simulink model "case7"  (R2024b)
settings: Solver=FixedStepAuto  StartTime=0  StopTime=1  FixedStep=1e-7  RelTol=1e-3
values from neighbouring files (symbols this model uses):
  SG_D_1_D = 0.01056    [IEEE9_case_parameters.m]    (also in case1_parameters.m; case2_parameters.m; case3_parameters.m; case4_parameters.m)
  SG_D_1_EnableSaturation = 0    [IEEE9_case_parameters.m]    (also in case1_parameters.m; case2_parameters.m; case3_parameters.m; case4_parameters.m)
  SG_D_1_f0 = 60    [IEEE9_case_parameters.m]    (also in case1_parameters.m; case2_parameters.m; case3_parameters.m; case4_parameters.m)
  SG_D_1_H = 7.5    [IEEE9_case_parameters.m]    (also in case1_parameters.m; case2_parameters.m; case3_parameters.m; case4_parameters.m)
  SG_D_1_K_A = 20    [IEEE9_case_parameters.m]    (also in case1_parameters.m; case2_parameters.m; case3_parameters.m; case4_parameters.m)
  SG_D_1_K_E = 1.000000e+1    (= 10)    [IEEE9_case_parameters.m]    (also in case1_parameters.m; case2_parameters.m; case3_parameters.m; case4_parameters.m)
  SG_D_1_K_F = 2.363    [IEEE9_case_parameters.m]    (also in case1_parameters.m; case2_parameters.m; case3_parameters.m; case4_parameters.m)
  SG_D_1_K_s = 0.5    [IEEE9_case_parameters.m]    (also in case1_parameters.m = 5; case2_parameters.m = 5; case3_parameters.m = 5; case4_parameters.m = 5)
  SG_D_1_R_a = 0.001088    [IEEE9_case_parameters.m]    (also in case1_parameters.m; case2_parameters.m; case3_parameters.m; case4_parameters.m)
  SG_D_1_S_A = 1    [IEEE9_case_parameters.m]    (also in case1_parameters.m; case2_parameters.m; case3_parameters.m; case4_parameters.m)
  SG_D_1_S_B = 0.103    [IEEE9_case_parameters.m]    (also in case1_parameters.m; case2_parameters.m; case3_parameters.m; case4_parameters.m)
  SG_D_1_S_N = 10.659857    [IEEE9_case_parameters.m]    (also in case1_parameters.m; case2_parameters.m; case3_parameters.m; case4_parameters.m)
  SG_D_1_SpeedPara = 200    [IEEE9_case_parameters.m]    (also in case1_parameters.m; case2_parameters.m; case3_parameters.m; case4_parameters.m)
  SG_D_1_T_0 = 0.720173    [IEEE9_case_parameters.m]    (also in case1_parameters.m = 0.755522; case2_parameters.m = 0.808931; case3_parameters.m = 0.869402; case4_parameters.m = 0.729316)
  SG_D_1_T_1 = 0.3    [IEEE9_case_parameters.m]    (also in case1_parameters.m; case2_parameters.m; case3_parameters.m; case4_parameters.m)
  SG_D_1_T_2 = 0.05    [IEEE9_case_parameters.m]    (also in case1_parameters.m; case2_parameters.m; case3_parameters.m; case4_parameters.m)
  SG_D_1_T_3 = 0.02    [IEEE9_case_parameters.m]    (also in case1_parameters.m; case2_parameters.m; case3_parameters.m; case4_parameters.m)
  SG_D_1_T_4 = 0.005    [IEEE9_case_parameters.m]    (also in case1_parameters.m; case2_parameters.m; case3_parameters.m; case4_parameters.m)
  SG_D_1_T_A = 0.02    [IEEE9_case_parameters.m]    (also in case1_parameters.m; case2_parameters.m; case3_parameters.m; case4_parameters.m)
  SG_D_1_T_dd = 8.000000e+0    (= 8)    [IEEE9_case_parameters.m]    (also in case1_parameters.m; case2_parameters.m; case3_parameters.m; case4_parameters.m)
  SG_D_1_T_ddd = 0.04    [IEEE9_case_parameters.m]    (also in case1_parameters.m; case2_parameters.m; case3_parameters.m; case4_parameters.m)
  SG_D_1_T_E = 0.314    [IEEE9_case_parameters.m]    (also in case1_parameters.m; case2_parameters.m; case3_parameters.m; case4_parameters.m)
  SG_D_1_T_F = 0.35    [IEEE9_case_parameters.m]    (also in case1_parameters.m; case2_parameters.m; case3_parameters.m; case4_parameters.m)
  SG_D_1_T_qd = 0.8    [IEEE9_case_parameters.m]    (also in case1_parameters.m; case2_parameters.m; case3_parameters.m; case4_parameters.m)
  SG_D_1_T_qdd = 0.02    [IEEE9_case_parameters.m]    (also in case1_parameters.m; case2_parameters.m; case3_parameters.m; case4_parameters.m)
  SG_D_1_T_speed = 0.1    [IEEE9_case_parameters.m]    (also in case1_parameters.m = 200; case2_parameters.m = 200; case3_parameters.m = 200; case4_parameters.m = 200)
  SG_D_1_T_w = 0.5    [IEEE9_case_parameters.m]    (also in case1_parameters.m; case2_parameters.m; case3_parameters.m; case4_parameters.m)
  SG_D_1_V_ref = 1.990276    [IEEE9_case_parameters.m]    (also in case1_parameters.m = 2.042296; case2_parameters.m = 2.051388; case3_parameters.m = 2.089584; case4_parameters.m = 2.01845)
  SG_D_1_w_ref = 376.991118    [IEEE9_case_parameters.m]    (also in case1_parameters.m; case2_parameters.m; case3_parameters.m; case4_parameters.m)
  SG_D_1_wb = 6.000000e+1    (= 60)    [IEEE9_case_parameters.m]    (also in case1_parameters.m; case2_parameters.m; case3_parameters.m; case4_parameters.m)
  SG_D_1_x_d = 1.9    [IEEE9_case_parameters.m]    (also in case1_parameters.m; case2_parameters.m; case3_parameters.m; case4_parameters.m)
  SG_D_1_x_dd = 0.302    [IEEE9_case_parameters.m]    (also in case1_parameters.m; case2_parameters.m; case3_parameters.m; case4_parameters.m)
  SG_D_1_x_ddd = 0.204    [IEEE9_case_parameters.m]    (also in case1_parameters.m; case2_parameters.m; case3_parameters.m; case4_parameters.m)
  SG_D_1_x_l = 0.05    [IEEE9_case_parameters.m]    (also in case1_parameters.m; case2_parameters.m; case3_parameters.m; case4_parameters.m)
  SG_D_1_x_q = 1.3    [IEEE9_case_parameters.m]    (also in case1_parameters.m; case2_parameters.m; case3_parameters.m; case4_parameters.m)
  SG_D_1_x_qd = 0.5    [IEEE9_case_parameters.m]    (also in case1_parameters.m; case2_parameters.m; case3_parameters.m; case4_parameters.m)
  SG_D_1_x_qdd = 0.3    [IEEE9_case_parameters.m]    (also in case1_parameters.m; case2_parameters.m; case3_parameters.m; case4_parameters.m)
  SG_D_2_D = 0.02    [IEEE9_case_parameters.m]    (also in case1_parameters.m; case2_parameters.m; case3_parameters.m; case4_parameters.m)
  SG_D_2_EnableSaturation = 0    [IEEE9_case_parameters.m]    (also in case1_parameters.m; case2_parameters.m; case3_parameters.m; case4_parameters.m)
  SG_D_2_f0 = 60    [IEEE9_case_parameters.m]    (also in case1_parameters.m; case2_parameters.m; case3_parameters.m; case4_parameters.m)
  SG_D_2_H = 8.000000e+0    (= 8)    [IEEE9_case_parameters.m]    (also in case1_parameters.m; case2_parameters.m; case3_parameters.m; case4_parameters.m)
  SG_D_2_K_A = 20    [IEEE9_case_parameters.m]    (also in case1_parameters.m; case2_parameters.m; case3_parameters.m; case4_parameters.m)
  SG_D_2_K_E = 1.000000e+1    (= 10)    [IEEE9_case_parameters.m]    (also in case1_parameters.m; case2_parameters.m; case3_parameters.m; case4_parameters.m)
  SG_D_2_K_F = 2.363    [IEEE9_case_parameters.m]    (also in case1_parameters.m; case2_parameters.m; case3_parameters.m; case4_parameters.m)
  SG_D_2_K_s = 0.5    [IEEE9_case_parameters.m]    (also in case1_parameters.m = 4; case2_parameters.m = 4; case3_parameters.m = 4; case4_parameters.m = 4)
  SG_D_2_R_a = 0.001088    [IEEE9_case_parameters.m]    (also in case1_parameters.m; case2_parameters.m; case3_parameters.m; case4_parameters.m)
  SG_D_2_S_A = 1    [IEEE9_case_parameters.m]    (also in case1_parameters.m; case2_parameters.m; case3_parameters.m; case4_parameters.m)
  SG_D_2_S_B = 0.103    [IEEE9_case_parameters.m]    (also in case1_parameters.m; case2_parameters.m; case3_parameters.m; case4_parameters.m)
  SG_D_2_S_N = 10.659857    [IEEE9_case_parameters.m]    (also in case1_parameters.m; case2_parameters.m; case3_parameters.m; case4_parameters.m)
  SG_D_2_SpeedPara = 200    [IEEE9_case_parameters.m]    (also in case1_parameters.m; case2_parameters.m; case3_parameters.m; case4_parameters.m)
  SG_D_2_T_0 = 1.632913    [IEEE9_case_parameters.m]    (also in case1_parameters.m = 1.632925; case2_parameters.m = 1.632915; case3_parameters.m = 1.632914; case4_parameters.m = 1.632927)
  SG_D_2_T_1 = 0.2    [IEEE9_case_parameters.m]    (also in case1_parameters.m; case2_parameters.m; case3_parameters.m; case4_parameters.m)
  SG_D_2_T_2 = 0.05    [IEEE9_case_parameters.m]    (also in case1_parameters.m; case2_parameters.m; case3_parameters.m; case4_parameters.m)
  SG_D_2_T_3 = 0.02    [IEEE9_case_parameters.m]    (also in case1_parameters.m; case2_parameters.m; case3_parameters.m; case4_parameters.m)
  SG_D_2_T_4 = 0.005    [IEEE9_case_parameters.m]    (also in case1_parameters.m; case2_parameters.m; case3_parameters.m; case4_parameters.m)
  SG_D_2_T_A = 0.02    [IEEE9_case_parameters.m]    (also in case1_parameters.m; case2_parameters.m; case3_parameters.m; case4_parameters.m)
  SG_D_2_T_dd = 7.9    [IEEE9_case_parameters.m]    (also in case1_parameters.m; case2_parameters.m; case3_parameters.m; case4_parameters.m)
  SG_D_2_T_ddd = 0.04    [IEEE9_case_parameters.m]    (also in case1_parameters.m; case2_parameters.m; case3_parameters.m; case4_parameters.m)
  SG_D_2_T_E = 0.314    [IEEE9_case_parameters.m]    (also in case1_parameters.m; case2_parameters.m; case3_parameters.m; case4_parameters.m)
  SG_D_2_T_F = 0.35    [IEEE9_case_parameters.m]    (also in case1_parameters.m; case2_parameters.m; case3_parameters.m; case4_parameters.m)
  SG_D_2_T_qd = 0.8    [IEEE9_case_parameters.m]    (also in case1_parameters.m; case2_parameters.m; case3_parameters.m; case4_parameters.m)
  SG_D_2_T_qdd = 0.015    [IEEE9_case_parameters.m]    (also in case1_parameters.m; case2_parameters.m; case3_parameters.m; case4_parameters.m)
  SG_D_2_T_speed = 0.1    [IEEE9_case_parameters.m]    (also in case1_parameters.m = 150; case2_parameters.m = 150; case3_parameters.m = 150; case4_parameters.m = 150)
  SG_D_2_T_w = 0.35    [IEEE9_case_parameters.m]    (also in case1_parameters.m; case2_parameters.m; case3_parameters.m; case4_parameters.m)
  SG_D_2_V_ref = 2.58547    [IEEE9_case_parameters.m]    (also in case1_parameters.m = 2.597896; case2_parameters.m = 2.587136; case3_parameters.m = 2.586042; case4_parameters.m = 2.599679)
  SG_D_2_w_ref = 376.991118    [IEEE9_case_parameters.m]    (also in case1_parameters.m; case2_parameters.m; case3_parameters.m; case4_parameters.m)
  SG_D_2_wb = 6.000000e+1    (= 60)    [IEEE9_case_parameters.m]    (also in case1_parameters.m; case2_parameters.m; case3_parameters.m; case4_parameters.m)
  SG_D_2_x_d = 1.8    [IEEE9_case_parameters.m]    (also in case1_parameters.m; case2_parameters.m; case3_parameters.m; case4_parameters.m)
  SG_D_2_x_dd = 0.302    [IEEE9_case_parameters.m]    (also in case1_parameters.m; case2_parameters.m; case3_parameters.m; case4_parameters.m)
  SG_D_2_x_ddd = 0.204    [IEEE9_case_parameters.m]    (also in case1_parameters.m; case2_parameters.m; case3_parameters.m; case4_parameters.m)
  SG_D_2_x_l = 0.05    [IEEE9_case_parameters.m]    (also in case1_parameters.m; case2_parameters.m; case3_parameters.m; case4_parameters.m)
  SG_D_2_x_q = 1.25    [IEEE9_case_parameters.m]    (also in case1_parameters.m; case2_parameters.m; case3_parameters.m; case4_parameters.m)
  SG_D_2_x_qd = 0.5    [IEEE9_case_parameters.m]    (also in case1_parameters.m; case2_parameters.m; case3_parameters.m; case4_parameters.m)
  SG_D_2_x_qdd = 0.3    [IEEE9_case_parameters.m]    (also in case1_parameters.m; case2_parameters.m; case3_parameters.m; case4_parameters.m)
  SG_D_3_D = 0.02    [IEEE9_case_parameters.m]    (also in case1_parameters.m; case2_parameters.m; case3_parameters.m; case4_parameters.m)
  SG_D_3_EnableSaturation = 0    [IEEE9_case_parameters.m]    (also in case1_parameters.m; case2_parameters.m; case3_parameters.m; case4_parameters.m)
  SG_D_3_f0 = 60    [IEEE9_case_parameters.m]    (also in case1_parameters.m; case2_parameters.m; case3_parameters.m; case4_parameters.m)
  SG_D_3_H = 7.7    [IEEE9_case_parameters.m]    (also in case1_parameters.m; case2_parameters.m; case3_parameters.m; case4_parameters.m)
  SG_D_3_K_A = 20    [IEEE9_case_parameters.m]    (also in case1_parameters.m; case2_parameters.m; case3_parameters.m; case4_parameters.m)
  SG_D_3_K_E = 1.000000e+1    (= 10)    [IEEE9_case_parameters.m]    (also in case1_parameters.m; case2_parameters.m; case3_parameters.m; case4_parameters.m)
  SG_D_3_K_F = 2.363    [IEEE9_case_parameters.m]    (also in case1_parameters.m; case2_parameters.m; case3_parameters.m; case4_parameters.m)
  SG_D_3_K_s = 0.2    [IEEE9_case_parameters.m]    (also in case1_parameters.m = 2; case2_parameters.m = 2; case3_parameters.m = 2; case4_parameters.m = 2)
  SG_D_3_R_a = 0.001088    [IEEE9_case_parameters.m]    (also in case1_parameters.m; case2_parameters.m; case3_parameters.m; case4_parameters.m)
  SG_D_3_S_A = 1    [IEEE9_case_parameters.m]    (also in case1_parameters.m; case2_parameters.m; case3_parameters.m; case4_parameters.m)
  SG_D_3_S_B = 0.103    [IEEE9_case_parameters.m]    (also in case1_parameters.m; case2_parameters.m; case3_parameters.m; case4_parameters.m)
  SG_D_3_S_N = 10.659857    [IEEE9_case_parameters.m]    (also in case1_parameters.m; case2_parameters.m; case3_parameters.m; case4_parameters.m)
  SG_D_3_SpeedPara = 200    [IEEE9_case_parameters.m]    (also in case1_parameters.m; case2_parameters.m; case3_parameters.m; case4_parameters.m)
  SG_D_3_T_0 = 0.850788    [IEEE9_case_parameters.m]    (also in case1_parameters.m = 0.850786; case2_parameters.m = 0.850787; case3_parameters.m; case4_parameters.m = 0.850786)
  SG_D_3_T_1 = 0.2    [IEEE9_case_parameters.m]    (also in case1_parameters.m; case2_parameters.m; case3_parameters.m; case4_parameters.m)
  SG_D_3_T_2 = 0.05    [IEEE9_case_parameters.m]    (also in case1_parameters.m; case2_parameters.m; case3_parameters.m; case4_parameters.m)
  SG_D_3_T_3 = 0.02    [IEEE9_case_parameters.m]    (also in case1_parameters.m; case2_parameters.m; case3_parameters.m; case4_parameters.m)
  SG_D_3_T_4 = 0.005    [IEEE9_case_parameters.m]    (also in case1_parameters.m; case2_parameters.m; case3_parameters.m; case4_parameters.m)
  SG_D_3_T_A = 0.02    [IEEE9_case_parameters.m]    (also in case1_parameters.m; case2_parameters.m; case3_parameters.m; case4_parameters.m)
  SG_D_3_T_dd = 8.1    [IEEE9_case_parameters.m]    (also in case1_parameters.m; case2_parameters.m; case3_parameters.m; case4_parameters.m)
  SG_D_3_T_ddd = 0.04    [IEEE9_case_parameters.m]    (also in case1_parameters.m; case2_parameters.m; case3_parameters.m; case4_parameters.m)
  SG_D_3_T_E = 0.314    [IEEE9_case_parameters.m]    (also in case1_parameters.m; case2_parameters.m; case3_parameters.m; case4_parameters.m)
  SG_D_3_T_F = 0.35    [IEEE9_case_parameters.m]    (also in case1_parameters.m; case2_parameters.m; case3_parameters.m; case4_parameters.m)
  SG_D_3_T_qd = 0.8    [IEEE9_case_parameters.m]    (also in case1_parameters.m; case2_parameters.m; case3_parameters.m; case4_parameters.m)
  SG_D_3_T_qdd = 0.015    [IEEE9_case_parameters.m]    (also in case1_parameters.m; case2_parameters.m; case3_parameters.m; case4_parameters.m)
  SG_D_3_T_speed = 0.1    [IEEE9_case_parameters.m]    (also in case1_parameters.m = 180; case2_parameters.m = 180; case3_parameters.m = 180; case4_parameters.m = 180)
  SG_D_3_T_w = 0.4    [IEEE9_case_parameters.m]    (also in case1_parameters.m; case2_parameters.m; case3_parameters.m; case4_parameters.m)
  SG_D_3_V_ref = 1.892727    [IEEE9_case_parameters.m]    (also in case1_parameters.m = 1.906439; case2_parameters.m = 1.895535; case3_parameters.m = 1.892105; case4_parameters.m = 1.906598)
  SG_D_3_w_ref = 376.991118    [IEEE9_case_parameters.m]    (also in case1_parameters.m; case2_parameters.m; case3_parameters.m; case4_parameters.m)
  SG_D_3_wb = 6.000000e+1    (= 60)    [IEEE9_case_parameters.m]    (also in case1_parameters.m; case2_parameters.m; case3_parameters.m; case4_parameters.m)
  SG_D_3_x_d = 1.85    [IEEE9_case_parameters.m]    (also in case1_parameters.m; case2_parameters.m; case3_parameters.m; case4_parameters.m)
  SG_D_3_x_dd = 0.302    [IEEE9_case_parameters.m]    (also in case1_parameters.m; case2_parameters.m; case3_parameters.m; case4_parameters.m)
  SG_D_3_x_ddd = 0.204    [IEEE9_case_parameters.m]    (also in case1_parameters.m; case2_parameters.m; case3_parameters.m; case4_parameters.m)
  SG_D_3_x_l = 0.05    [IEEE9_case_parameters.m]    (also in case1_parameters.m; case2_parameters.m; case3_parameters.m; case4_parameters.m)
  SG_D_3_x_q = 1.2    [IEEE9_case_parameters.m]    (also in case1_parameters.m; case2_parameters.m; case3_parameters.m; case4_parameters.m)
  SG_D_3_x_qd = 0.5    [IEEE9_case_parameters.m]    (also in case1_parameters.m; case2_parameters.m; case3_parameters.m; case4_parameters.m)
  SG_D_3_x_qdd = 0.3    [IEEE9_case_parameters.m]    (also in case1_parameters.m; case2_parameters.m; case3_parameters.m; case4_parameters.m)
(part 11 of 12)

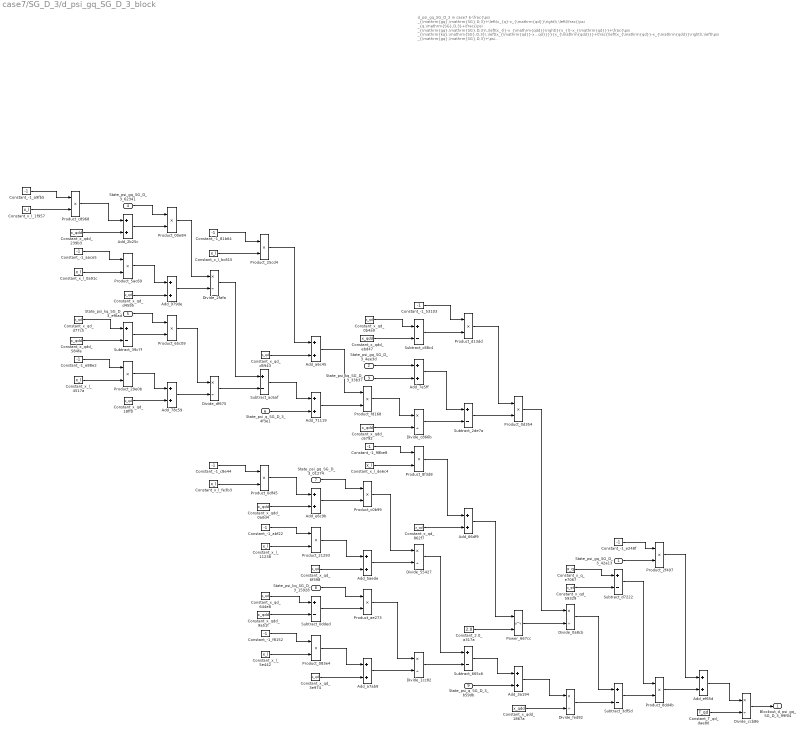
== system case7/SG_D_3/d_psi_gq_SG_D_3_block ==
  note: d_psi_gq_SG_D_3 in case7
      | $-\frac{\psi _{\mathrm{gq},\mathrm{SG},D,3}+\left(x_{q}-x_{\mathrm{qd}}\right)\,\left(\frac{\psi _{q,\mathrm{SG},D,3}+\frac{\psi _{\mathrm{gq},\mathrm{SG},D,3}\,\left(x_{l}-x_{\mathrm{qdd}}\right)}{x_{l}-x_{\mathrm{qd}}}+\frac{\psi _{\mathrm{kq},\mathrm{SG},D,3}\,\left(x_{\mathrm{qd}}-x_{\mathrm{qdd}}\right)}{x_{l}-x_{\mathrm{qd}}}}{x_{\mathrm{qdd}}}+\frac{\left(x_{\mathrm{qd}}-x_{\mathrm{qdd}}\right)\,\left(\psi _{\mathrm{gq},\mathrm{SG},D,3}+\psi _{\mathrm{kq},\mathrm{SG},D,3}+\frac{\left(x_{l}-x_{\mathrm{qd}}\right)\,\left(\psi _{q,\mathrm{SG},D,3}+\frac{\psi _{\mathrm{gq},\mathrm{SG},D,3}\,\left(x_{l}-x_{\mathrm{qdd}}\right)}{x_{l}-x_{\mathrm{qd}}}+\frac{\psi _{\mathrm{kq},\mathrm{SG},D,3}\,\left(x_{\mathrm{qd}}-x_{\mathrm{qdd}}\right)}{x_{l}-x_{\mathrm{qd}}}\right)}{x_{\mathrm{qdd}}}\right)}{{\left(x_{l}-x_{\mathrm{qd}}\right)}^2}\right)}{T_{\mathrm{qd}}}$
      | Automatically generated on 2025-10-31 19:25:57 .
  State_psi_gq_SG_D_3_42a13 : Inport
  State_psi_gq_SG_D_3_4ee3d : Inport  Port=2
  State_psi_kq_SG_D_3_33b37 : Inport  Port=3
  State_psi_gq_SG_D_3_62341 : Inport  Port=4
  State_psi_kq_SG_D_3_ef6ad : Inport  Port=5
  State_psi_q_SG_D_3_4f3e1 : Inport  Port=6
  State_psi_gq_SG_D_3_01274 : Inport  Port=7
  State_psi_kq_SG_D_3_15928 : Inport  Port=8
  State_psi_q_SG_D_3_b59db : Inport  Port=9
  Add_2b25c : Sum
  Add_3a194 : Sum
  Add_5aede : Sum
  Add_66df9 : Sum
  Add_71119 : Sum
  Add_78c59 : Sum
  Add_7e5ff : Sum
  Add_979de : Sum
  Add_a6c45 : Sum
  Add_a7ab9 : Sum
  Add_e6c9b : Sum
  Add_ef65d : Sum
  Constant_-1_53103 : Constant  Value=-1
  Constant_-1_81b64 : Constant  Value=-1
  Constant_-1_98be8 : Constant  Value=-1
  Constant_-1_a9fb5 : Constant  Value=-1
  Constant_-1_aace5 : Constant  Value=-1
  Constant_-1_abf22 : Constant  Value=-1
  Constant_-1_c8e44 : Constant  Value=-1
  Constant_-1_e248f : Constant  Value=-1
  Constant_-1_e88e2 : Constant  Value=-1
  Constant_-1_f8152 : Constant  Value=-1
  Constant_2.0_a317a : Constant  Value=2.0
  Constant_T_qd_dae80 : Constant  Value=T_qd
  Constant_x_l_0a91c : Constant  Value=x_l
  Constant_x_l_11238 : Constant  Value=x_l
  Constant_x_l_1f957 : Constant  Value=x_l
  Constant_x_l_4517a : Constant  Value=x_l
  Constant_x_l_5e442 : Constant  Value=x_l
  Constant_x_l_bc815 : Constant  Value=x_l
  Constant_x_l_de6c4 : Constant  Value=x_l
  Constant_x_l_fe3b3 : Constant  Value=x_l
  Constant_x_q_e7067 : Constant  Value=x_q
  Constant_x_qd_0b4a9 : Constant  Value=x_qd
  Constant_x_qd_18ff0 : Constant  Value=x_qd
  Constant_x_qd_3e974 : Constant  Value=x_qd
  Constant_x_qd_59329 : Constant  Value=x_qd
  Constant_x_qd_644e8 : Constant  Value=x_qd
  Constant_x_qd_6f398 : Constant  Value=x_qd
  Constant_x_qd_862f7 : Constant  Value=x_qd
  Constant_x_qd_d4595 : Constant  Value=x_qd
  Constant_x_qd_d5943 : Constant  Value=x_qd
  Constant_x_qd_d77c5 : Constant  Value=x_qd
  Constant_x_qdd_0a0d4 : Constant  Value=x_qdd
  Constant_x_qdd_1867a : Constant  Value=x_qdd
  Constant_x_qdd_239b3 : Constant  Value=x_qdd
  Constant_x_qdd_584fa : Constant  Value=x_qdd
  Constant_x_qdd_9a51f : Constant  Value=x_qdd
  Constant_x_qdd_c6792 : Constant  Value=x_qdd
  Constant_x_qdd_ebd47 : Constant  Value=x_qdd
  Divide_0a8cb : Product  Inputs=*/
  Divide_1cc82 : Product  Inputs=*/
  Divide_2fafa : Product  Inputs=*/
  Divide_55427 : Product  Inputs=*/
  Divide_c866b : Product  Inputs=*/
  Divide_ccb86 : Product  Inputs=*/
  Divide_df675 : Product  Inputs=*/
  Divide_fed82 : Product  Inputs=*/
  Power_667cc : Math  Operator=pow
  Product_00e84 : Product
  Product_083e4 : Product
  Product_0d354 : Product
  Product_0df45 : Product
  Product_21293 : Product
  Product_25cd4 : Product
  Product_29e0b : Product
  Product_2f497 : Product
  Product_5ac69 : Product
  Product_65c09 : Product
  Product_8dd4b : Product
  Product_8f3d8 : Product
  Product_ae273 : Product
  Product_c0b99 : Product
  Product_c8968 : Product
  Product_d13dd : Product
  Product_fd168 : Product
  Subtract_0dded : Sum  Inputs=+-
  Subtract_2de7a : Sum  Inputs=+-
  Subtract_39c7f : Sum  Inputs=+-
  Subtract_3df5d : Sum  Inputs=+-
  Subtract_665c6 : Sum  Inputs=+-
  Subtract_ac6af : Sum  Inputs=+-
  Subtract_c88c4 : Sum  Inputs=+-
  Subtract_d7222 : Sum  Inputs=+-
  Blockout_d_psi_gq_SG_D_3_99f04 : Outport
  wires:
  Constant_x_l_de6c4/1 -> Product_8f3d8/2
  Constant_x_qd_d77c5/1 -> Subtract_39c7f/1
  Add_a6c45/1 -> Product_fd168/1
  Constant_-1_a9fb5/1 -> Product_c8968/1
  Add_2b25c/1 -> Product_00e84/2
  Constant_x_qdd_584fa/1 -> Subtract_39c7f/2
  Constant_x_qd_d5943/1 -> Add_a6c45/2
  Constant_x_l_1f957/1 -> Product_c8968/2
  Constant_x_l_0a91c/1 -> Product_5ac69/2
  Add_a7ab9/1 -> Divide_1cc82/2
  State_psi_kq_SG_D_3_33b37/1 -> Add_7e5ff/2
  Constant_x_qdd_239b3/1 -> Add_2b25c/2
  Product_c8968/1 -> Add_2b25c/1
  Constant_x_qd_3e974/1 -> Add_a7ab9/2
  Product_d13dd/1 -> Product_0d354/1
  Constant_-1_c8e44/1 -> Product_0df45/1
  Constant_-1_aace5/1 -> Product_5ac69/1
  Constant_-1_e88e2/1 -> Product_29e0b/1
  Constant_x_l_4517a/1 -> Product_29e0b/2
  Constant_-1_53103/1 -> Product_d13dd/1
  Constant_-1_e248f/1 -> Product_2f497/1
  State_psi_gq_SG_D_3_62341/1 -> Product_00e84/1
  Product_0df45/1 -> Add_e6c9b/1
  Product_5ac69/1 -> Add_979de/1
  Product_083e4/1 -> Add_a7ab9/1
  Constant_x_qd_d4595/1 -> Add_979de/2
  Constant_-1_abf22/1 -> Product_21293/1
  State_psi_kq_SG_D_3_ef6ad/1 -> Product_65c09/1
  Subtract_39c7f/1 -> Product_65c09/2
  Product_29e0b/1 -> Add_78c59/1
  Add_e6c9b/1 -> Product_c0b99/2
  Add_979de/1 -> Divide_2fafa/2
  Constant_x_qd_18ff0/1 -> Add_78c59/2
  Product_00e84/1 -> Divide_2fafa/1
  Constant_T_qd_dae80/1 -> Divide_ccb86/2
  Product_21293/1 -> Add_5aede/1
  Product_65c09/1 -> Divide_df675/1
  Product_ae273/1 -> Divide_1cc82/1
  Add_78c59/1 -> Divide_df675/2
  Constant_-1_81b64/1 -> Product_25cd4/1
  Constant_x_qdd_c6792/1 -> Divide_c866b/2
  Constant_x_l_bc815/1 -> Product_25cd4/2
  Divide_2fafa/1 -> Subtract_ac6af/1
  Constant_x_qd_59329/1 -> Subtract_d7222/2
  Add_5aede/1 -> Divide_55427/2
  Divide_df675/1 -> Subtract_ac6af/2
  Constant_x_l_fe3b3/1 -> Product_0df45/2
  Product_25cd4/1 -> Add_a6c45/1
  Constant_-1_98be8/1 -> Product_8f3d8/1
  Constant_x_l_11238/1 -> Product_21293/2
  Subtract_ac6af/1 -> Add_71119/1
  State_psi_q_SG_D_3_4f3e1/1 -> Add_71119/2
  Constant_-1_f8152/1 -> Product_083e4/1
  Constant_x_qdd_0a0d4/1 -> Add_e6c9b/2
  Constant_x_qd_644e8/1 -> Subtract_0dded/1
  Constant_x_qdd_9a51f/1 -> Subtract_0dded/2
  Constant_x_l_5e442/1 -> Product_083e4/2
  Add_71119/1 -> Product_fd168/2
  Constant_x_qdd_ebd47/1 -> Subtract_c88c4/2
  State_psi_gq_SG_D_3_01274/1 -> Product_c0b99/1
  Constant_x_qd_6f398/1 -> Add_5aede/2
  Divide_0a8cb/1 -> Subtract_3df5d/1
  State_psi_kq_SG_D_3_15928/1 -> Product_ae273/1
  Subtract_0dded/1 -> Product_ae273/2
  Constant_x_qd_0b4a9/1 -> Subtract_c88c4/1
  State_psi_gq_SG_D_3_4ee3d/1 -> Add_7e5ff/1
  Product_fd168/1 -> Divide_c866b/1
  Product_c0b99/1 -> Divide_55427/1
  Subtract_c88c4/1 -> Product_d13dd/2
  Add_7e5ff/1 -> Subtract_2de7a/1
  Divide_c866b/1 -> Subtract_2de7a/2
  Product_8f3d8/1 -> Add_66df9/1
  Constant_x_qd_862f7/1 -> Add_66df9/2
  Divide_55427/1 -> Subtract_665c6/1
  Divide_1cc82/1 -> Subtract_665c6/2
  Subtract_2de7a/1 -> Product_0d354/2
  Add_66df9/1 -> Power_667cc/1
  Constant_2.0_a317a/1 -> Power_667cc/2
  Subtract_665c6/1 -> Add_3a194/1
  State_psi_q_SG_D_3_b59db/1 -> Add_3a194/2
  Product_0d354/1 -> Divide_0a8cb/1
  Power_667cc/1 -> Divide_0a8cb/2
  Add_3a194/1 -> Divide_fed82/1
  Constant_x_qdd_1867a/1 -> Divide_fed82/2
  Constant_x_q_e7067/1 -> Subtract_d7222/1
  Divide_fed82/1 -> Subtract_3df5d/2
  State_psi_gq_SG_D_3_42a13/1 -> Product_2f497/2
  Subtract_d7222/1 -> Product_8dd4b/1
  Subtract_3df5d/1 -> Product_8dd4b/2
  Product_2f497/1 -> Add_ef65d/1
  Product_8dd4b/1 -> Add_ef65d/2
  Add_ef65d/1 -> Divide_ccb86/1
  Divide_ccb86/1 -> Blockout_d_psi_gq_SG_D_3_99f04/1

== system case7/SG_D_3/d_psi_kq_SG_D_3_block ==
  note: d_psi_kq_SG_D_3 in case7
      | $-\frac{\psi _{\mathrm{gq},\mathrm{SG},D,3}+\psi _{\mathrm{kq},\mathrm{SG},D,3}+\frac{\left(x_{l}-x_{\mathrm{qd}}\right)\,\left(\psi _{q,\mathrm{SG},D,3}+\frac{\psi _{\mathrm{gq},\mathrm{SG},D,3}\,\left(x_{l}-x_{\mathrm{qdd}}\right)}{x_{l}-x_{\mathrm{qd}}}+\frac{\psi _{\mathrm{kq},\mathrm{SG},D,3}\,\left(x_{\mathrm{qd}}-x_{\mathrm{qdd}}\right)}{x_{l}-x_{\mathrm{qd}}}\right)}{x_{\mathrm{qdd}}}}{T_{\mathrm{qdd}}}$
      | Automatically generated on 2025-10-31 19:25:58 .
  State_psi_gq_SG_D_3_cecd3 : Inport
  State_psi_kq_SG_D_3_60998 : Inport  Port=2
  State_psi_gq_SG_D_3_2a36c : Inport  Port=3
  State_psi_kq_SG_D_3_904ed : Inport  Port=4
  State_psi_q_SG_D_3_3b0fa : Inport  Port=5
  Add_14141 : Sum
  Add_5f367 : Sum
  Add_7b92b : Sum
  Add_88eea : Sum
  Add_8f67f : Sum
  Add_e8599 : Sum
  Constant_-1_03dcc : Constant  Value=-1
  Constant_-1_07b11 : Constant  Value=-1
  Constant_-1_3317b : Constant  Value=-1
  Constant_-1_5726a : Constant  Value=-1
  Constant_-1_8191a : Constant  Value=-1
  Constant_T_qdd_a084b : Constant  Value=T_qdd
  Constant_x_l_0fefe : Constant  Value=x_l
  Constant_x_l_50fdd : Constant  Value=x_l
  Constant_x_l_6da91 : Constant  Value=x_l
  Constant_x_l_af22f : Constant  Value=x_l
  Constant_x_qd_37301 : Constant  Value=x_qd
  Constant_x_qd_5f0e4 : Constant  Value=x_qd
  Constant_x_qd_5f42d : Constant  Value=x_qd
  Constant_x_qd_c0782 : Constant  Value=x_qd
  Constant_x_qdd_4207d : Constant  Value=x_qdd
  Constant_x_qdd_4f5d6 : Constant  Value=x_qdd
  Constant_x_qdd_66940 : Constant  Value=x_qdd
  Divide_0bd73 : Product  Inputs=*/
  Divide_863c3 : Product  Inputs=*/
  Divide_b3fe8 : Product  Inputs=*/
  Divide_b9d21 : Product  Inputs=*/
  Product_0c19d : Product
  Product_47df6 : Product
  Product_595ce : Product
  Product_63cb6 : Product
  Product_8259f : Product
  Product_a25e8 : Product
  Product_e1e2e : Product
  Product_fcb12 : Product
  Subtract_3a63e : Sum  Inputs=+-
  Subtract_73cb7 : Sum  Inputs=+-
  Subtract_96d2b : Sum  Inputs=+-
  Blockout_d_psi_kq_SG_D_3_d1c2e : Outport
  wires:
  State_psi_q_SG_D_3_3b0fa/1 -> Add_8f67f/2
  Constant_-1_3317b/1 -> Product_8259f/1
  Constant_-1_07b11/1 -> Product_0c19d/1
  Constant_-1_5726a/1 -> Product_e1e2e/1
  Constant_x_l_af22f/1 -> Product_8259f/2
  Constant_x_qdd_66940/1 -> Add_14141/2
  Product_47df6/1 -> Add_e8599/1
  Constant_x_l_50fdd/1 -> Product_0c19d/2
  Constant_x_qd_37301/1 -> Subtract_3a63e/1
  Product_0c19d/1 -> Add_14141/1
  Constant_x_l_6da91/1 -> Product_63cb6/2
  Constant_x_qdd_4207d/1 -> Subtract_3a63e/2
  Constant_-1_03dcc/1 -> Product_47df6/1
  Constant_x_l_0fefe/1 -> Product_47df6/2
  State_psi_gq_SG_D_3_2a36c/1 -> Product_595ce/1
  Add_14141/1 -> Product_595ce/2
  Add_8f67f/1 -> Product_a25e8/2
  Product_8259f/1 -> Add_7b92b/1
  Constant_x_qd_5f42d/1 -> Add_7b92b/2
  State_psi_kq_SG_D_3_904ed/1 -> Product_fcb12/1
  Subtract_3a63e/1 -> Product_fcb12/2
  Add_7b92b/1 -> Divide_b9d21/2
  Constant_x_qd_c0782/1 -> Add_e8599/2
  Product_595ce/1 -> Divide_b9d21/1
  Product_fcb12/1 -> Divide_b3fe8/1
  Add_e8599/1 -> Divide_b3fe8/2
  Constant_-1_8191a/1 -> Product_63cb6/1
  Divide_b9d21/1 -> Subtract_73cb7/1
  Add_88eea/1 -> Divide_0bd73/1
  Divide_b3fe8/1 -> Subtract_73cb7/2
  Divide_0bd73/1 -> Blockout_d_psi_kq_SG_D_3_d1c2e/1
  Product_63cb6/1 -> Add_5f367/1
  Constant_x_qd_5f0e4/1 -> Add_5f367/2
  Subtract_73cb7/1 -> Add_8f67f/1
  State_psi_gq_SG_D_3_cecd3/1 -> Product_e1e2e/2
  Add_5f367/1 -> Product_a25e8/1
  Constant_T_qdd_a084b/1 -> Divide_0bd73/2
  Product_e1e2e/1 -> Subtract_96d2b/1
  State_psi_kq_SG_D_3_60998/1 -> Subtract_96d2b/2
  Product_a25e8/1 -> Divide_863c3/1
  Constant_x_qdd_4f5d6/1 -> Divide_863c3/2
  Subtract_96d2b/1 -> Add_88eea/1
  Divide_863c3/1 -> Add_88eea/2

== system case7/SG_D_3/d_psi_q_SG_D_3_block ==
  note: d_psi_q_SG_D_3 in case7
      | $2\,\pi \,f_{0}\,\left(v_{d,\mathrm{SG},D,3}\,\cos\left(\theta _{\mathrm{SG},D,3}\right)+v_{q,\mathrm{SG},D,3}\,\sin\left(\theta _{\mathrm{SG},D,3}\right)-\frac{R_{a}\,\left(\psi _{q,\mathrm{SG},D,3}+\frac{\psi _{\mathrm{gq},\mathrm{SG},D,3}\,\left(x_{l}-x_{\mathrm{qdd}}\right)}{x_{l}-x_{\mathrm{qd}}}+\frac{\psi _{\mathrm{kq},\mathrm{SG},D,3}\,\left(x_{\mathrm{qd}}-x_{\mathrm{qdd}}\right)}{x_{l}-x_{\mathrm{qd}}}\right)}{x_{\mathrm{qdd}}}-\frac{\psi _{d,\mathrm{SG},D,3}\,w_{\mathrm{SG},D,3}}{2\,f_{0}\,\pi }\right)$
      | Automatically generated on 2025-10-31 19:25:41 .
  State_psi_gq_SG_D_3_f880b : Inport
  State_psi_kq_SG_D_3_940c9 : Inport  Port=2
  State_psi_q_SG_D_3_7fdb8 : Inport  Port=3
  Input_v_d_SG_D_3_f4c2d : Inport  Port=4
  State_theta_SG_D_3_e0e57 : Inport  Port=5
  Input_v_q_SG_D_3_303a8 : Inport  Port=6
  State_theta_SG_D_3_98ce1 : Inport  Port=7
  State_psi_d_SG_D_3_074a8 : Inport  Port=8
  State_w_SG_D_3_e996e : Inport  Port=9
  Add_3c206 : Sum
  Add_5eab2 : Sum
  Add_6e5a4 : Sum
  Add_bb9a2 : Sum
  Add_fab3a : Sum
  Constant_-1_828c4 : Constant  Value=-1
  Constant_-1_dada7 : Constant  Value=-1
  Constant_-1_eab26 : Constant  Value=-1
  Constant_-2.0_2aa60 : Constant  Value=-2.0
  Constant_2.0_c8072 : Constant  Value=2.0
  Constant_R_a_502e2 : Constant  Value=R_a
  Constant_f0_45527 : Constant  Value=f0
  Constant_f0_afd4c : Constant  Value=f0
  Constant_pi_e6714 : Constant  Value=pi
  Constant_pi_e7b35 : Constant  Value=pi
  Constant_x_l_62e6d : Constant  Value=x_l
  Constant_x_l_74d75 : Constant  Value=x_l
  Constant_x_l_d22a4 : Constant  Value=x_l
  Constant_x_qd_ada06 : Constant  Value=x_qd
  Constant_x_qd_d568d : Constant  Value=x_qd
  Constant_x_qd_f9ca8 : Constant  Value=x_qd
  Constant_x_qdd_17ffd : Constant  Value=x_qdd
  Constant_x_qdd_8f833 : Constant  Value=x_qdd
  Constant_x_qdd_aa089 : Constant  Value=x_qdd
  Divide_15d08 : Product  Inputs=*/
  Divide_25346 : Product  Inputs=*/
  Divide_2b0e5 : Product  Inputs=*/
  Divide_de1e9 : Product  Inputs=*/
  MathFunc_cos_21777 : Trigonometry  Operator=cos
  MathFunc_sin_e5274 : Trigonometry
  Product_1ab73 : Product
  Product_1cf76 : Product
  Product_5428b : Product
  Product_6640f : Product
  Product_837c1 : Product
  Product_90474 : Product
  Product_b1ffa : Product
  Product_bba8c : Product
  Product_bfb7a : Product
  Product_c1af3 : Product
  Product_d4398 : Product
  Product_ea4d3 : Product
  Product_f7cba : Product
  Product_fcd8c : Product
  Subtract_126e3 : Sum  Inputs=+-
  Subtract_14233 : Sum  Inputs=+-
  Subtract_24a11 : Sum  Inputs=+-
  Subtract_eb27b : Sum  Inputs=+-
  Blockout_d_psi_q_SG_D_3_20592 : Outport
  wires:
  Constant_x_qd_f9ca8/1 -> Subtract_126e3/1
  Constant_pi_e6714/1 -> Product_bba8c/2
  Product_5428b/1 -> Divide_25346/1
  Constant_x_l_d22a4/1 -> Product_f7cba/2
  Constant_f0_afd4c/1 -> Product_d4398/2
  State_w_SG_D_3_e996e/1 -> Product_1cf76/2
  Constant_-1_dada7/1 -> Product_1ab73/1
  Constant_x_qdd_aa089/1 -> Add_3c206/2
  Input_v_d_SG_D_3_f4c2d/1 -> Product_ea4d3/1
  Constant_x_qdd_8f833/1 -> Subtract_126e3/2
  Constant_x_l_74d75/1 -> Product_1ab73/2
  Divide_de1e9/1 -> Add_6e5a4/2
  Product_1ab73/1 -> Add_3c206/1
  Constant_2.0_c8072/1 -> Product_bba8c/1
  Add_5eab2/1 -> Product_5428b/2
  Constant_-1_828c4/1 -> Product_f7cba/1
  Constant_x_qd_d568d/1 -> Add_bb9a2/2
  Constant_-1_eab26/1 -> Product_c1af3/1
  Subtract_eb27b/1 -> Subtract_14233/1
  Constant_x_l_62e6d/1 -> Product_c1af3/2
  Subtract_14233/1 -> Add_6e5a4/1
  Constant_f0_45527/1 -> Product_fcd8c/2
  State_theta_SG_D_3_98ce1/1 -> MathFunc_sin_e5274/1
  Constant_x_qd_ada06/1 -> Add_fab3a/2
  State_psi_gq_SG_D_3_f880b/1 -> Product_837c1/1
  Add_3c206/1 -> Product_837c1/2
  Product_bba8c/1 -> Product_fcd8c/1
  Product_f7cba/1 -> Add_fab3a/1
  State_psi_kq_SG_D_3_940c9/1 -> Product_90474/1
  Subtract_126e3/1 -> Product_90474/2
  Product_c1af3/1 -> Add_bb9a2/1
  MathFunc_sin_e5274/1 -> Product_6640f/2
  Product_837c1/1 -> Divide_15d08/1
  Product_fcd8c/1 -> Divide_de1e9/2
  Add_fab3a/1 -> Divide_15d08/2
  Product_90474/1 -> Divide_2b0e5/1
  Add_bb9a2/1 -> Divide_2b0e5/2
  Input_v_q_SG_D_3_303a8/1 -> Product_6640f/1
  Divide_15d08/1 -> Subtract_24a11/1
  Subtract_24a11/1 -> Add_5eab2/1
  Divide_2b0e5/1 -> Subtract_24a11/2
  Divide_25346/1 -> Subtract_eb27b/1
  State_psi_q_SG_D_3_7fdb8/1 -> Add_5eab2/2
  Product_6640f/1 -> Subtract_14233/2
  Constant_R_a_502e2/1 -> Product_5428b/1
  State_theta_SG_D_3_e0e57/1 -> MathFunc_cos_21777/1
  Constant_x_qdd_17ffd/1 -> Divide_25346/2
  MathFunc_cos_21777/1 -> Product_ea4d3/2
  Constant_-2.0_2aa60/1 -> Product_b1ffa/1
  Product_ea4d3/1 -> Subtract_eb27b/2
  State_psi_d_SG_D_3_074a8/1 -> Product_1cf76/1
  Constant_pi_e7b35/1 -> Product_b1ffa/2
  Product_1cf76/1 -> Divide_de1e9/1
  Product_b1ffa/1 -> Product_d4398/1
  Product_d4398/1 -> Product_bfb7a/1
  Add_6e5a4/1 -> Product_bfb7a/2
  Product_bfb7a/1 -> Blockout_d_psi_q_SG_D_3_20592/1

== system case7/SG_D_3/d_theta_SG_D_3_block ==
  note: d_theta_SG_D_3 in case7
      | $w_{\mathrm{SG},D,3}-2\,\pi \,f_{0}$
      | Automatically generated on 2025-10-31 19:26:02 .
  State_w_SG_D_3_e06ca : Inport
  Add_bb76a : Sum
  Constant_-2.0_1ba68 : Constant  Value=-2.0
  Constant_f0_936f8 : Constant  Value=f0
  Constant_pi_c22b3 : Constant  Value=pi
  Product_4b4d3 : Product
  Product_5b9a2 : Product
  Blockout_d_theta_SG_D_3_abfc2 : Outport
  wires:
  Constant_-2.0_1ba68/1 -> Product_4b4d3/1
  Constant_pi_c22b3/1 -> Product_4b4d3/2
  State_w_SG_D_3_e06ca/1 -> Add_bb76a/2
  Product_4b4d3/1 -> Product_5b9a2/1
  Constant_f0_936f8/1 -> Product_5b9a2/2
  Product_5b9a2/1 -> Add_bb76a/1
  Add_bb76a/1 -> Blockout_d_theta_SG_D_3_abfc2/1

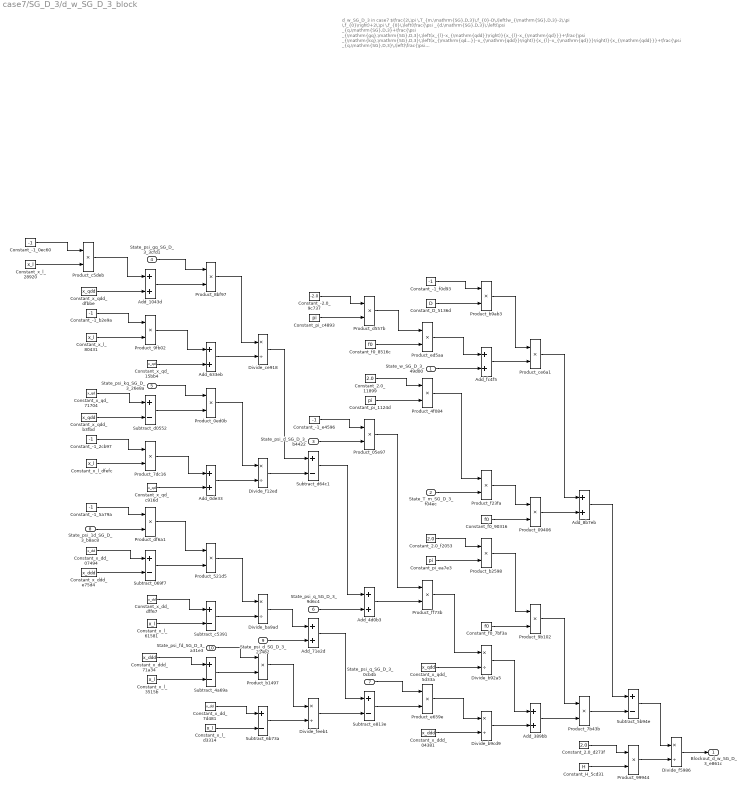
== system case7/SG_D_3/d_w_SG_D_3_block ==
  note: d_w_SG_D_3 in case7
      | $\frac{2\,\pi \,T_{m,\mathrm{SG},D,3}\,f_{0}-D\,\left(w_{\mathrm{SG},D,3}-2\,\pi \,f_{0}\right)+2\,\pi \,f_{0}\,\left(\frac{\psi _{d,\mathrm{SG},D,3}\,\left(\psi _{q,\mathrm{SG},D,3}+\frac{\psi _{\mathrm{gq},\mathrm{SG},D,3}\,\left(x_{l}-x_{\mathrm{qdd}}\right)}{x_{l}-x_{\mathrm{qd}}}+\frac{\psi _{\mathrm{kq},\mathrm{SG},D,3}\,\left(x_{\mathrm{qd}}-x_{\mathrm{qdd}}\right)}{x_{l}-x_{\mathrm{qd}}}\right)}{x_{\mathrm{qdd}}}+\frac{\psi _{q,\mathrm{SG},D,3}\,\left(\frac{\psi _{\mathrm{1d},\mathrm{SG},D,3}\,\left(x_{\mathrm{dd}}-x_{\mathrm{ddd}}\right)}{x_{\mathrm{dd}}-x_{l}}-\psi _{d,\mathrm{SG},D,3}+\frac{\psi _{\mathrm{fd},\mathrm{SG},D,3}\,\left(x_{\mathrm{ddd}}-x_{l}\right)}{x_{\mathrm{dd}}-x_{l}}\right)}{x_{\mathrm{ddd}}}\right)}{2\,H}$
      | Automatically generated on 2025-10-31 19:26:00 .
  State_w_SG_D_3_49d00 : Inport
  State_T_m_SG_D_3_f04ec : Inport  Port=2
  State_psi_d_SG_D_3_b4422 : Inport  Port=3
  State_psi_gq_SG_D_3_3cfd1 : Inport  Port=4
  State_psi_kq_SG_D_3_26e8a : Inport  Port=5
  State_psi_q_SG_D_3_9d6c4 : Inport  Port=6
  State_psi_q_SG_D_3_0cb4b : Inport  Port=7
  State_psi_1d_SG_D_3_b8ac8 : Inport  Port=8
  State_psi_d_SG_D_3_21482 : Inport  Port=9
  State_psi_fd_SG_D_3_a31e3 : Inport  Port=10
  Add_0de33 : Sum
  Add_1043d : Sum
  Add_389bb : Sum
  Add_4d0b3 : Sum
  Add_633eb : Sum
  Add_71e2d : Sum
  Add_8b7eb : Sum
  Add_fc4f5 : Sum
  Constant_-1_0ec60 : Constant  Value=-1
  Constant_-1_2cb97 : Constant  Value=-1
  Constant_-1_5a79a : Constant  Value=-1
  Constant_-1_b2e9a : Constant  Value=-1
  Constant_-1_e4596 : Constant  Value=-1
  Constant_-1_f0d93 : Constant  Value=-1
  Constant_-2.0_9c737 : Constant  Value=-2.0
  Constant_2.0_11899 : Constant  Value=2.0
  Constant_2.0_d273f : Constant  Value=2.0
  Constant_2.0_f2053 : Constant  Value=2.0
  Constant_D_5136d : Constant  Value=D
  Constant_H_5cd31 : Constant  Value=H
  Constant_f0_7bf3a : Constant  Value=f0
  Constant_f0_8516c : Constant  Value=f0
  Constant_f0_90316 : Constant  Value=f0
  Constant_pi_1124d : Constant  Value=pi
  Constant_pi_c4893 : Constant  Value=pi
  Constant_pi_ea7e3 : Constant  Value=pi
  Constant_x_dd_07494 : Constant  Value=x_dd
  Constant_x_dd_7d481 : Constant  Value=x_dd
  Constant_x_dd_dff67 : Constant  Value=x_dd
  Constant_x_ddd_04381 : Constant  Value=x_ddd
  Constant_x_ddd_71a34 : Constant  Value=x_ddd
  Constant_x_ddd_e75d4 : Constant  Value=x_ddd
  Constant_x_l_28920 : Constant  Value=x_l
  Constant_x_l_3515b : Constant  Value=x_l
  Constant_x_l_61581 : Constant  Value=x_l
  Constant_x_l_80431 : Constant  Value=x_l
  Constant_x_l_d3314 : Constant  Value=x_l
  Constant_x_l_dfefc : Constant  Value=x_l
  Constant_x_qd_15bb4 : Constant  Value=x_qd
  Constant_x_qd_71704 : Constant  Value=x_qd
  Constant_x_qd_c916d : Constant  Value=x_qd
  Constant_x_qdd_5d33a : Constant  Value=x_qdd
  Constant_x_qdd_b3fbd : Constant  Value=x_qdd
  Constant_x_qdd_dfbbe : Constant  Value=x_qdd
  Divide_b92a5 : Product  Inputs=*/
  Divide_b9cd9 : Product  Inputs=*/
  Divide_ba9ad : Product  Inputs=*/
  Divide_ce918 : Product  Inputs=*/
  Divide_f12ed : Product  Inputs=*/
  Divide_f5986 : Product  Inputs=*/
  Divide_feeb1 : Product  Inputs=*/
  Product_05e97 : Product
  Product_09406 : Product
  Product_0ed0b : Product
  Product_4f084 : Product
  Product_521d5 : Product
  Product_7b43b : Product
  Product_7dc16 : Product
  Product_8bf97 : Product
  Product_99944 : Product
  Product_9b102 : Product
  Product_9fb02 : Product
  Product_b1497 : Product
  Product_b2598 : Product
  Product_b9ab3 : Product
  Product_c5deb : Product
  Product_ce6a1 : Product
  Product_d557b : Product
  Product_df6a1 : Product
  Product_e659e : Product
  Product_ed5aa : Product
  Product_f23fa : Product
  Product_ff73b : Product
  Subtract_069f7 : Sum  Inputs=+-
  Subtract_4a69a : Sum  Inputs=+-
  Subtract_5b94e : Sum  Inputs=+-
  Subtract_6b73a : Sum  Inputs=+-
  Subtract_c5391 : Sum  Inputs=+-
  Subtract_d0552 : Sum  Inputs=+-
  Subtract_d64c1 : Sum  Inputs=+-
  Subtract_e813e : Sum  Inputs=+-
  Blockout_d_w_SG_D_3_e861c : Outport
  wires:
  Constant_x_qd_71704/1 -> Subtract_d0552/1
  Subtract_069f7/1 -> Product_521d5/2
  Subtract_5b94e/1 -> Divide_f5986/1
  Constant_-1_0ec60/1 -> Product_c5deb/1
  Add_1043d/1 -> Product_8bf97/2
  Constant_x_qdd_b3fbd/1 -> Subtract_d0552/2
  Subtract_4a69a/1 -> Product_b1497/2
  Constant_x_l_28920/1 -> Product_c5deb/2
  State_psi_d_SG_D_3_21482/1 -> Add_71e2d/2
  Add_633eb/1 -> Divide_ce918/2
  Constant_x_dd_dff67/1 -> Subtract_c5391/1
  Constant_x_l_80431/1 -> Product_9fb02/2
  Constant_-1_f0d93/1 -> Product_b9ab3/1
  Divide_feeb1/1 -> Subtract_e813e/2
  Constant_x_ddd_e75d4/1 -> Subtract_069f7/2
  Constant_x_qdd_dfbbe/1 -> Add_1043d/2
  Constant_pi_1124d/1 -> Product_4f084/2
  Product_c5deb/1 -> Add_1043d/1
  Constant_-2.0_9c737/1 -> Product_d557b/1
  Constant_-1_b2e9a/1 -> Product_9fb02/1
  Constant_2.0_f2053/1 -> Product_b2598/1
  Product_d557b/1 -> Product_ed5aa/1
  Constant_-1_2cb97/1 -> Product_7dc16/1
  Subtract_d64c1/1 -> Add_4d0b3/1
  Constant_x_l_dfefc/1 -> Product_7dc16/2
  Constant_x_l_3515b/1 -> Subtract_4a69a/2
  Constant_-1_5a79a/1 -> Product_df6a1/1
  State_psi_1d_SG_D_3_b8ac8/1 -> Product_df6a1/2
  Constant_x_dd_07494/1 -> Subtract_069f7/1
  Product_df6a1/1 -> Product_521d5/1
  State_psi_gq_SG_D_3_3cfd1/1 -> Product_8bf97/1
  Constant_x_qd_15bb4/1 -> Add_633eb/2
  Product_9fb02/1 -> Add_633eb/1
  State_psi_kq_SG_D_3_26e8a/1 -> Product_0ed0b/1
  Subtract_d0552/1 -> Product_0ed0b/2
  Product_b2598/1 -> Product_9b102/1
  Product_ed5aa/1 -> Add_fc4f5/1
  Product_7dc16/1 -> Add_0de33/1
  State_psi_q_SG_D_3_0cb4b/1 -> Product_e659e/1
  Constant_x_qd_c916d/1 -> Add_0de33/2
  Constant_x_l_61581/1 -> Subtract_c5391/2
  Constant_x_ddd_71a34/1 -> Subtract_4a69a/1
  Constant_x_l_d3314/1 -> Subtract_6b73a/2
  Product_8bf97/1 -> Divide_ce918/1
  Product_0ed0b/1 -> Divide_f12ed/1
  Add_0de33/1 -> Divide_f12ed/2
  Product_521d5/1 -> Divide_ba9ad/1
  Subtract_c5391/1 -> Divide_ba9ad/2
  Constant_2.0_11899/1 -> Product_4f084/1
  State_psi_fd_SG_D_3_a31e3/1 -> Product_b1497/1
  Constant_x_dd_7d481/1 -> Subtract_6b73a/1
  Divide_ce918/1 -> Subtract_d64c1/1
  Product_b1497/1 -> Divide_feeb1/1
  Divide_f12ed/1 -> Subtract_d64c1/2
  Divide_ba9ad/1 -> Add_71e2d/1
  Product_7b43b/1 -> Subtract_5b94e/2
  Subtract_6b73a/1 -> Divide_feeb1/2
  Constant_pi_c4893/1 -> Product_d557b/2
  Constant_pi_ea7e3/1 -> Product_b2598/2
  Constant_-1_e4596/1 -> Product_05e97/1
  State_psi_d_SG_D_3_b4422/1 -> Product_05e97/2
  State_psi_q_SG_D_3_9d6c4/1 -> Add_4d0b3/2
  Add_71e2d/1 -> Subtract_e813e/1
  Constant_f0_8516c/1 -> Product_ed5aa/2
  Product_05e97/1 -> Product_ff73b/1
  Add_4d0b3/1 -> Product_ff73b/2
  Subtract_e813e/1 -> Product_e659e/2
  Constant_D_5136d/1 -> Product_b9ab3/2
  State_w_SG_D_3_49d00/1 -> Add_fc4f5/2
  Product_4f084/1 -> Product_f23fa/1
  State_T_m_SG_D_3_f04ec/1 -> Product_f23fa/2
  Product_ff73b/1 -> Divide_b92a5/1
  Constant_x_qdd_5d33a/1 -> Divide_b92a5/2
  Product_e659e/1 -> Divide_b9cd9/1
  Constant_x_ddd_04381/1 -> Divide_b9cd9/2
  Product_b9ab3/1 -> Product_ce6a1/1
  Add_fc4f5/1 -> Product_ce6a1/2
  Product_f23fa/1 -> Product_09406/1
  Constant_f0_90316/1 -> Product_09406/2
  Constant_f0_7bf3a/1 -> Product_9b102/2
  Divide_b92a5/1 -> Add_389bb/1
  Divide_b9cd9/1 -> Add_389bb/2
  Product_ce6a1/1 -> Add_8b7eb/1
  Product_09406/1 -> Add_8b7eb/2
  Product_9b102/1 -> Product_7b43b/1
  Add_389bb/1 -> Product_7b43b/2
  Add_8b7eb/1 -> Subtract_5b94e/1
  Constant_2.0_d273f/1 -> Product_99944/1
  Constant_H_5cd31/1 -> Product_99944/2
  Product_99944/1 -> Divide_f5986/2
  Divide_f5986/1 -> Blockout_d_w_SG_D_3_e861c/1

== system case7/SG_D_3/i_d_SG_D_3_block ==
  note: i_d_SG_D_3 in case7
      | $\frac{\sin\left(\theta _{\mathrm{SG},D,3}\right)\,\left(\frac{\psi _{\mathrm{1d},\mathrm{SG},D,3}\,\left(x_{\mathrm{dd}}-x_{\mathrm{ddd}}\right)}{x_{\mathrm{dd}}-x_{l}}-\psi _{d,\mathrm{SG},D,3}+\frac{\psi _{\mathrm{fd},\mathrm{SG},D,3}\,\left(x_{\mathrm{ddd}}-x_{l}\right)}{x_{\mathrm{dd}}-x_{l}}\right)}{x_{\mathrm{ddd}}}-\frac{\cos\left(\theta _{\mathrm{SG},D,3}\right)\,\left(\psi _{q,\mathrm{SG},D,3}+\frac{\psi _{\mathrm{gq},\mathrm{SG},D,3}\,\left(x_{l}-x_{\mathrm{qdd}}\right)}{x_{l}-x_{\mathrm{qd}}}+\frac{\psi _{\mathrm{kq},\mathrm{SG},D,3}\,\left(x_{\mathrm{qd}}-x_{\mathrm{qdd}}\right)}{x_{l}-x_{\mathrm{qd}}}\right)}{x_{\mathrm{qdd}}}$
      | Automatically generated on 2025-10-31 19:26:28 .
  State_psi_gq_SG_D_3_6922b : Inport
  State_psi_kq_SG_D_3_f6ce0 : Inport  Port=2
  State_psi_q_SG_D_3_af60f : Inport  Port=3
  State_theta_SG_D_3_14959 : Inport  Port=4
  State_psi_1d_SG_D_3_0e0c9 : Inport  Port=5
  State_psi_d_SG_D_3_94a65 : Inport  Port=6
  State_psi_fd_SG_D_3_81ff2 : Inport  Port=7
  State_theta_SG_D_3_4b034 : Inport  Port=8
  Add_3388b : Sum
  Add_72f5d : Sum
  Add_c8fb3 : Sum
  Add_ec535 : Sum
  Add_f25bb : Sum
  Constant_-1_0388b : Constant  Value=-1
  Constant_-1_10056 : Constant  Value=-1
  Constant_-1_31b05 : Constant  Value=-1
  Constant_-1_9e46f : Constant  Value=-1
  Constant_-1_f32e6 : Constant  Value=-1
  Constant_x_dd_28ab8 : Constant  Value=x_dd
  Constant_x_dd_8a86a : Constant  Value=x_dd
  Constant_x_dd_e79a7 : Constant  Value=x_dd
  Constant_x_ddd_2b022 : Constant  Value=x_ddd
  Constant_x_ddd_5cd9a : Constant  Value=x_ddd
  Constant_x_ddd_78bcf : Constant  Value=x_ddd
  Constant_x_l_4baca : Constant  Value=x_l
  Constant_x_l_7a528 : Constant  Value=x_l
  Constant_x_l_87f02 : Constant  Value=x_l
  Constant_x_l_b7a67 : Constant  Value=x_l
  Constant_x_l_e1022 : Constant  Value=x_l
  Constant_x_l_ed596 : Constant  Value=x_l
  Constant_x_qd_15473 : Constant  Value=x_qd
  Constant_x_qd_76fd0 : Constant  Value=x_qd
  Constant_x_qd_ec6e2 : Constant  Value=x_qd
  Constant_x_qdd_83307 : Constant  Value=x_qdd
  Constant_x_qdd_b5470 : Constant  Value=x_qdd
  Constant_x_qdd_d244e : Constant  Value=x_qdd
  Divide_2a1c5 : Product  Inputs=*/
  Divide_540bc : Product  Inputs=*/
  Divide_5b84e : Product  Inputs=*/
  Divide_a4956 : Product  Inputs=*/
  Divide_c3b97 : Product  Inputs=*/
  Divide_ea9e2 : Product  Inputs=*/
  MathFunc_cos_0d010 : Trigonometry  Operator=cos
  MathFunc_sin_aff6c : Trigonometry
  Product_1dcd1 : Product
  Product_3123c : Product
  Product_322c8 : Product
  Product_4a43e : Product
  Product_5af64 : Product
  Product_9802b : Product
  Product_9c629 : Product
  Product_bfc65 : Product
  Product_c8751 : Product
  Product_d775b : Product
  Product_e1d38 : Product
  Subtract_3cb63 : Sum  Inputs=+-
  Subtract_4442c : Sum  Inputs=+-
  Subtract_4ab5a : Sum  Inputs=+-
  Subtract_55765 : Sum  Inputs=+-
  Subtract_6ef6c : Sum  Inputs=+-
  Subtract_9812f : Sum  Inputs=+-
  Subtract_9e9b8 : Sum  Inputs=+-
  Subtract_db903 : Sum  Inputs=+-
  Blockout_i_d_SG_D_3_97111 : Outport
  wires:
  Constant_x_qd_ec6e2/1 -> Subtract_55765/1
  Subtract_db903/1 -> Blockout_i_d_SG_D_3_97111/1
  Constant_-1_10056/1 -> Product_c8751/1
  Constant_x_l_e1022/1 -> Product_1dcd1/2
  Constant_x_qdd_d244e/1 -> Add_ec535/2
  Constant_x_qdd_b5470/1 -> Subtract_55765/2
  Constant_x_l_7a528/1 -> Product_c8751/2
  Divide_a4956/1 -> Subtract_db903/1
  Product_c8751/1 -> Add_ec535/1
  Constant_x_ddd_2b022/1 -> Subtract_4ab5a/2
  Constant_-1_31b05/1 -> Product_1dcd1/1
  Constant_-1_0388b/1 -> Product_bfc65/1
  Constant_x_l_b7a67/1 -> Product_bfc65/2
  State_psi_1d_SG_D_3_0e0c9/1 -> Product_322c8/2
  State_psi_gq_SG_D_3_6922b/1 -> Product_9802b/1
  Product_322c8/1 -> Product_d775b/1
  Add_ec535/1 -> Product_9802b/2
  Product_1dcd1/1 -> Add_f25bb/1
  Constant_x_qd_15473/1 -> Add_f25bb/2
  State_psi_kq_SG_D_3_f6ce0/1 -> Product_9c629/1
  Subtract_6ef6c/1 -> Divide_c3b97/2
  Subtract_55765/1 -> Product_9c629/2
  Product_bfc65/1 -> Add_3388b/1
  Constant_x_ddd_78bcf/1 -> Subtract_4442c/1
  Constant_x_qd_76fd0/1 -> Add_3388b/2
  Constant_-1_9e46f/1 -> Product_322c8/1
  Constant_x_dd_e79a7/1 -> Subtract_4ab5a/1
  Product_9802b/1 -> Divide_5b84e/1
  Add_f25bb/1 -> Divide_5b84e/2
  Product_9c629/1 -> Divide_ea9e2/1
  Add_3388b/1 -> Divide_ea9e2/2
  Divide_c3b97/1 -> Subtract_9812f/2
  Subtract_4ab5a/1 -> Product_d775b/2
  State_theta_SG_D_3_14959/1 -> MathFunc_cos_0d010/1
  Constant_x_dd_28ab8/1 -> Subtract_9e9b8/1
  Product_e1d38/1 -> Product_3123c/1
  Constant_x_l_ed596/1 -> Subtract_9e9b8/2
  Add_72f5d/1 -> Subtract_9812f/1
  Constant_x_l_4baca/1 -> Subtract_4442c/2
  State_theta_SG_D_3_4b034/1 -> MathFunc_sin_aff6c/1
  Divide_5b84e/1 -> Subtract_3cb63/1
  Add_c8fb3/1 -> Product_e1d38/2
  Divide_ea9e2/1 -> Subtract_3cb63/2
  Product_d775b/1 -> Divide_540bc/1
  Subtract_9e9b8/1 -> Divide_540bc/2
  State_psi_fd_SG_D_3_81ff2/1 -> Product_5af64/1
  Divide_2a1c5/1 -> Subtract_db903/2
  Subtract_4442c/1 -> Product_5af64/2
  Constant_x_dd_8a86a/1 -> Subtract_6ef6c/1
  Subtract_3cb63/1 -> Add_c8fb3/1
  Constant_x_l_87f02/1 -> Subtract_6ef6c/2
  Constant_-1_f32e6/1 -> Product_e1d38/1
  State_psi_q_SG_D_3_af60f/1 -> Add_c8fb3/2
  Divide_540bc/1 -> Add_72f5d/1
  State_psi_d_SG_D_3_94a65/1 -> Add_72f5d/2
  Product_5af64/1 -> Divide_c3b97/1
  MathFunc_cos_0d010/1 -> Product_3123c/2
  MathFunc_sin_aff6c/1 -> Product_4a43e/2
  Subtract_9812f/1 -> Product_4a43e/1
  Product_3123c/1 -> Divide_a4956/1
  Constant_x_qdd_83307/1 -> Divide_a4956/2
  Product_4a43e/1 -> Divide_2a1c5/1
  Constant_x_ddd_5cd9a/1 -> Divide_2a1c5/2
